simulink model "Q4EQ2"  (R2026a)
settings: Solver=VariableStepAuto
settings Model: VariantFading=off

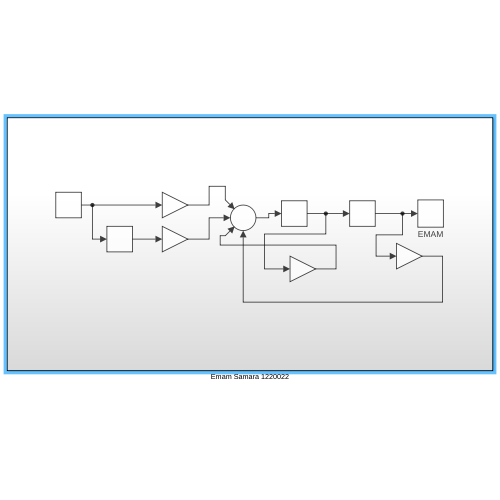
[thumbnail: Simulink's stored preview of the top-level diagram]
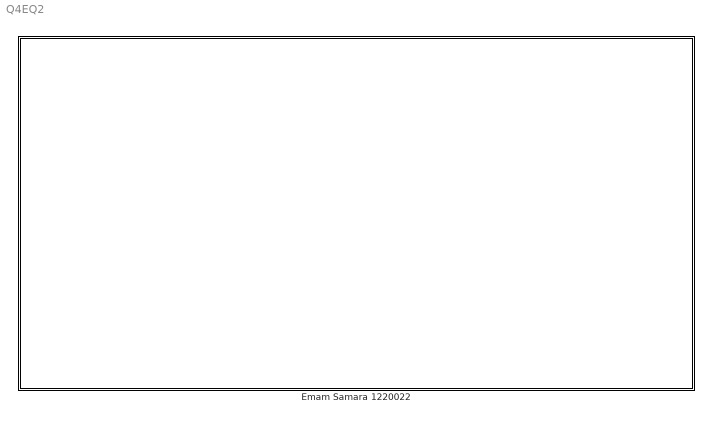
== system Q4EQ2 ==
  Emam Samara 1220022 : Subsystem

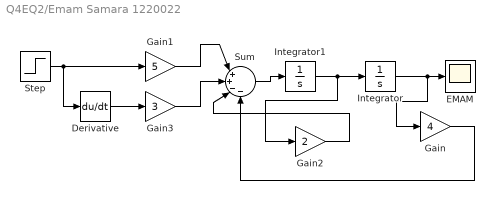
== system Q4EQ2/Emam Samara 1220022 ==
  Derivative : Derivative
  EMAM : Scope
      settings: ActiveDisplayYMinimum=-5.805666872429228  ActiveDisplayYMaximum=5.2451252113363456
  Gain : Gain  Gain=4
  Gain1 : Gain  Gain=5
  Gain2 : Gain  Gain=2
  Gain3 : Gain  Gain=3
  Integrator : Integrator
  Integrator1 : Integrator
  Step : Step  SampleTime=0
  Sum : Sum  Inputs=|++--
  wires:
  Step/1 -> Derivative/1, Gain1/1
  Gain3/1 -> Sum/2
  Gain2/1 -> Sum/3
  Integrator/1 -> Gain/1, EMAM/1
  Gain1/1 -> Sum/1
  Derivative/1 -> Gain3/1
  Sum/1 -> Integrator1/1
  Gain/1 -> Sum/4
  Integrator1/1 -> Gain2/1, Integrator/1
